simulink model "VDPOL"  (Simulink 10.0)
settings: Solver=ode45  StartTime=0.0  StopTime=10.0  RelTol=1e-3  EnableMultiTasking=on
settings Model: Creator=tjohnson  LastModifiedBy=unknown
settings DataIOCC: LimitDataPoints=on
settings DebuggingCC: UnderspecifiedInitializationDetection=Simplified  MergeDetectMultiDrivingBlocksExec=error
settings GRTTargetCC: GeneratePreprocessorConditionals=Disable all  CombineOutputUpdateFcns=on  GRTInterface=off
settings ConfigComp: CovExternalEMLEnable=off

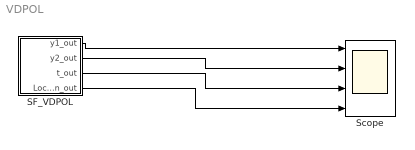
== system VDPOL ==
  SF_VDPOL : Stateflow chart  TreatAsAtomicUnit=on
  Scope : Scope  NumInputPorts=4
  wires:
  SF_VDPOL/1(y1_out) -> Scope/1
  SF_VDPOL/2(y2_out) -> Scope/2
  SF_VDPOL/3(t_out) -> Scope/3
  SF_VDPOL/4(Location_out) -> Scope/4

== stateflow chart SF_VDPOL ==
  settings: updateMethod=CONTINUOUS
  state VDPOL
    du:
    y1_dot = y2;
    y2_dot = k * (1.0 - y1 ^ 2.0) * y2 - y1;
    t_dot = 1.0;
    y1_out=y1;
    y2_out=y2;
    t_out=t;
    Location_out =1;
  (default) -> VDPOL : {t = 0.0; y1 = 2.0; y2 = 0.0;}
  data: k constant double =1000; stop_time constant double =2000; y1 local double; y1_out output double; y2 local double; y2_out output double; t local double; t_out output double; Location_out output double
  data y1 settings: updateMethod=SF_CONTINUOUS_TIME_DATA
  data y2 settings: updateMethod=SF_CONTINUOUS_TIME_DATA
  data t settings: updateMethod=SF_CONTINUOUS_TIME_DATA
